simulink model "dlbsTestHarnessDenseLayer"  (R2025b)
settings: Solver=VariableStepAuto  StartTime=0.0  StopTime=10.0  RelTol=1e-3
undefined symbols (not defined in the file or in its folder): b, dY, W, X
libraries: dlbsBlockExtractGradientGF x3, dlbsBlockDenseLayer x1, dlbsBlockInsertGradientGF x1
settings Model: Creator=lt6037  LastModifiedBy=lt6037

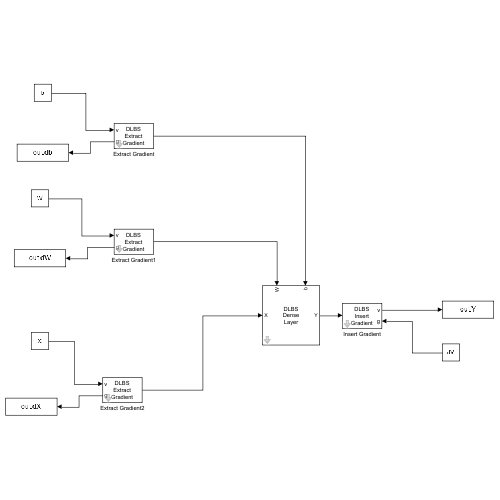
[thumbnail: Simulink's stored preview of the top-level diagram]
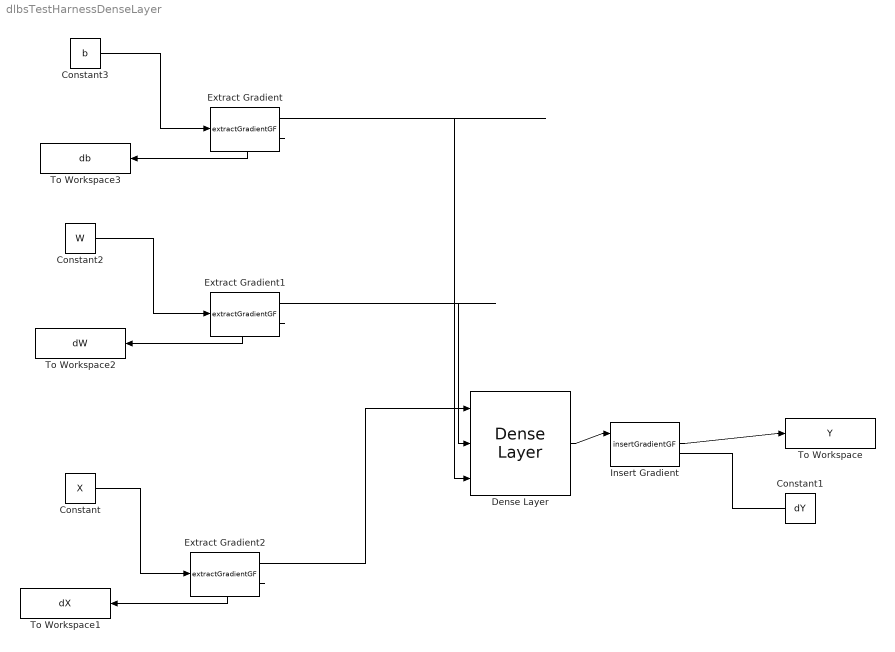
== system dlbsTestHarnessDenseLayer ==
  Constant : Constant  Value=X  VectorParams1D=off
  Constant1 : Constant  Value=dY  VectorParams1D=off
  Constant2 : Constant  Value=W  VectorParams1D=off
  Constant3 : Constant  Value=b  VectorParams1D=off
  Dense Layer : dlbsBlockDenseLayer/Dense Layer
  Extract Gradient : dlbsBlockExtractGradientGF/extractGradientGF
  Extract Gradient1 : dlbsBlockExtractGradientGF/extractGradientGF
  Extract Gradient2 : dlbsBlockExtractGradientGF/extractGradientGF
  Insert Gradient : dlbsBlockInsertGradientGF/insertGradientGF
  To Workspace : ToWorkspace  VariableName=Y  SaveFormat=Timeseries  SampleTime=-1
      settings: MaxDataPoints=1
  To Workspace1 : ToWorkspace  VariableName=dX  SaveFormat=Timeseries  SampleTime=-1
      settings: MaxDataPoints=1
  To Workspace2 : ToWorkspace  VariableName=dW  SaveFormat=Timeseries  SampleTime=-1
      settings: MaxDataPoints=1
  To Workspace3 : ToWorkspace  VariableName=db  SaveFormat=Timeseries  SampleTime=-1
      settings: MaxDataPoints=1
  wires:
  Extract Gradient2/2 -> To Workspace1/1
  Constant/1 -> Extract Gradient2/1
  Extract Gradient1/2 -> To Workspace2/1
  Constant2/1 -> Extract Gradient1/1
  Extract Gradient/2 -> To Workspace3/1
  Constant3/1 -> Extract Gradient/1
  Extract Gradient2/1 -> Dense Layer/1
  Extract Gradient1/1 -> Dense Layer/2
  Extract Gradient/1 -> Dense Layer/3
  Dense Layer/1 -> Insert Gradient/1
  Constant1/1 -> Insert Gradient/2
  Insert Gradient/1 -> To Workspace/1
